simulink subsystem "MPC6_nlpsol"  (R2022b)
settings: Solver=VariableStepAuto  StartTime=0.0  StopTime=10.0  RelTol=1e-3
undefined symbols (not defined in the file): param_global, param_MPC6, param_robot, param_weight_init
settings Model: Creator=emu  LastModifiedBy=emu
settings OptimizationCC: ReuseModelBlockBuffer=on

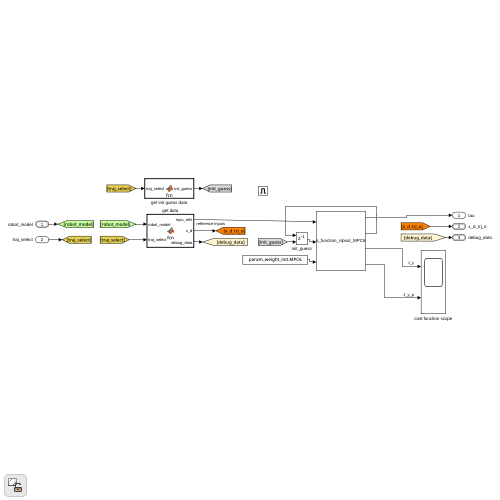
[thumbnail: Simulink's stored preview of the top-level diagram]
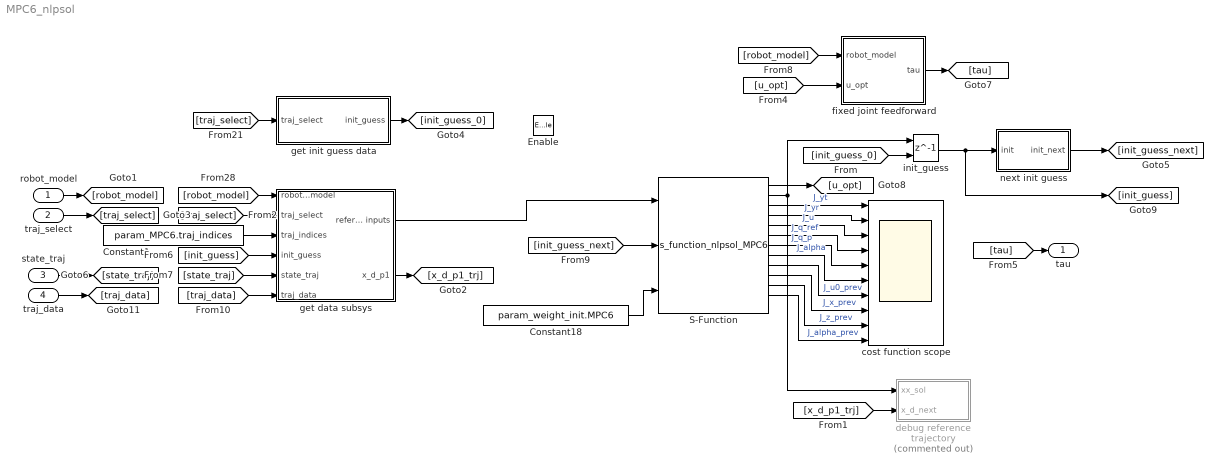
== system MPC6_nlpsol ==
  robot_model : Inport  OutDataTypeStr=Bus: robot_model
  traj_select : Inport  Port=2
  state_traj : Inport  Port=3  OutDataTypeStr=Bus: state_traj_bus
  traj_data : Inport  Port=4  OutDataTypeStr=Bus: traj_data_bus
  Enable : EnablePort
  Constant1 : Constant  Value=param_MPC6.traj_indices
  Constant18 : Constant  Value=param_weight_init.MPC6  VectorParams1D=off
  S-Function : S-Function  FunctionName=s_function_nlpsol_MPC6  Parameters='s_functions/fr3_no_hand_6dof/MPC6.casadi', 'MPC6'  SFunctionModules='MPC6'  SFunctionDeploymentMode=off  EnableBusSupport=off
  cost function scope : Scope  NumInputPorts=10
  debug reference trajectory : Subsystem  Commented=on
  fixed joint feedforward : MATLAB Function  TreatAsAtomicUnit=on
  get data subsys : Subsystem
  get init guess data : MATLAB Function  TreatAsAtomicUnit=on
  init_guess : Delay  DelayLength=1  InitialConditionSource=Input port  InitialCondition=1
      settings: InputPortMap=u0,p4
  next init guess : MATLAB Function  TreatAsAtomicUnit=on
  tau : Outport
  wires:
  S-Function/12 -> cost function scope/10  "J_alpha_prev"
  S-Function/7 -> cost function scope/5  "J_q_p"
  S-Function/10 -> cost function scope/8  "J_x_prev"
  S-Function/3 -> cost function scope/1  "J_yt"
  S-Function/6 -> cost function scope/4  "J_q_ref"
  S-Function/4 -> cost function scope/2  "J_yr"
  S-Function/5 -> cost function scope/3  "J_u"
  S-Function/11 -> cost function scope/9  "J_z_prev"
  S-Function/9 -> cost function scope/7  "J_u0_prev"
  S-Function/8 -> cost function scope/6  "J_alpha"
  next init guess/1(init_next) -> [init_guess_next]
  [init_guess_0] -> init_guess/2
  get init guess data/1(init_guess) -> [init_guess_0]
  S-Function/2 -> init_guess/1, debug reference trajectory/1(xx_sol)
  [traj_select] -> get init guess data/1(traj_select)
  traj_select/1 -> [traj_select]
  robot_model/1 -> [robot_model]
  Constant18/1 -> S-Function/3
  [x_d_p1_trj] -> debug reference trajectory/2(x_d_next)
  [robot_model] -> get data subsys/1(robot_model)
  [traj_select] -> get data subsys/2(traj_select)
  Constant1/1 -> get data subsys/3(traj_indices)
  get data subsys/1(reference inputs) -> S-Function/1
  get data subsys/2(x_d_p1) -> [x_d_p1_trj]
  state_traj/1 -> [state_traj]
  [state_traj] -> get data subsys/5(state_traj)
  fixed joint feedforward/1(tau) -> [tau]
  [robot_model] -> fixed joint feedforward/1(robot_model)
  [u_opt] -> fixed joint feedforward/2(u_opt)
  S-Function/1 -> [u_opt]
  [tau] -> tau/1
  init_guess/1 -> next init guess/1(init), [init_guess]
  [init_guess] -> get data subsys/4(init_guess)
  [init_guess_next] -> S-Function/2
  traj_data/1 -> [traj_data]
  [traj_data] -> get data subsys/6(traj_data)

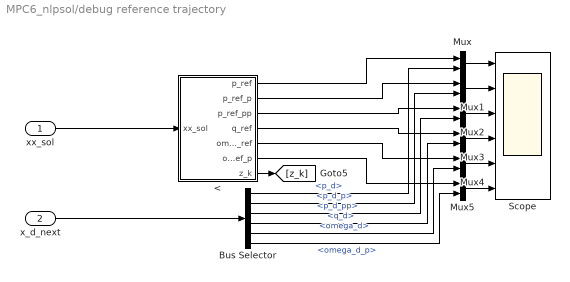
== system MPC6_nlpsol/debug reference trajectory ==
  xx_sol : Inport
  x_d_next : Inport  Port=2  OutDataTypeStr=Bus: x_d
  < : MATLAB Function  TreatAsAtomicUnit=on
  Bus Selector : BusSelector  OutputSignals=p_d,p_d_p,p_d_pp,q_d,omega_d,omega_d_p
  Mux{,1..5} (6 alike) : Mux  Inputs=2
  Scope : Scope  NumInputPorts=6
  wires:
  Mux1/1 -> Scope/2
  </3(p_ref_pp) -> Mux2/1
  Mux5/1 -> Scope/6
  Bus Selector/1 -> Mux/2  "<p_d>"
  Mux3/1 -> Scope/4
  Mux2/1 -> Scope/3
  Bus Selector/6 -> Mux5/2  "<omega_d_p>"
  </4(q_ref) -> Mux3/1
  Bus Selector/2 -> Mux1/2  "<p_d_p>"
  x_d_next/1 -> Bus Selector/1
  Mux/1 -> Scope/1
  </6(omega_ref_p) -> Mux5/1
  Bus Selector/4 -> Mux3/2  "<q_d>"
  </2(p_ref_p) -> Mux1/1
  </7(z_k) -> [z_k]
  </1(p_ref) -> Mux/1
  Bus Selector/5 -> Mux4/2  "<omega_d>"
  xx_sol/1 -> </1(xx_sol)
  </5(omega_ref) -> Mux4/1
  Bus Selector/3 -> Mux2/2  "<p_d_pp>"
  Mux4/1 -> Scope/5

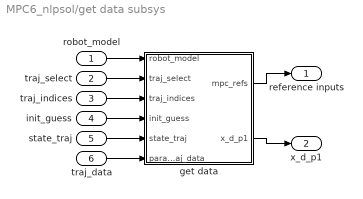
== system MPC6_nlpsol/get data subsys ==
  robot_model : Inport  OutDataTypeStr=Bus: robot_model
  traj_select : Inport  Port=2
  traj_indices : Inport  Port=3
  init_guess : Inport  Port=4
  state_traj : Inport  Port=5  OutDataTypeStr=Bus: state_traj_bus
  traj_data : Inport  Port=6  OutDataTypeStr=Bus: traj_data_bus
  get data : MATLAB Function  TreatAsAtomicUnit=on
  reference inputs : Outport
  x_d_p1 : Outport  Port=2  OutDataTypeStr=Bus: x_d
  wires:
  traj_data/1 -> get data/6(param_traj_data)
  init_guess/1 -> get data/4(init_guess)
  state_traj/1 -> get data/5(state_traj)
  traj_indices/1 -> get data/3(traj_indices)
  get data/1(mpc_refs) -> reference inputs/1
  robot_model/1 -> get data/1(robot_model)
  get data/2(x_d_p1) -> x_d_p1/1
  traj_select/1 -> get data/2(traj_select)

== matlab function MPC6_nlpsol/fixed joint feedforward ==
  data: robot_model input Bus: robot_model; tau output; u_opt input; param_robot parameter
function  tau = fcn(robot_model, u_opt, param_robot)

n = param_robot.n_DOF;

if size(u_opt, 2) ~= 0 && size(u_opt, 1) ~= 1
    n_indices = param_robot.n_indices;
    n_red = param_robot.n_red;

    tau_red = u_opt(1:n_red);
    %q_d_pp = u_opt(1+n_red:2*n_red);

    M = robot_model.M;      % inertia matrix
    g = robot_model.g;
    C_rnea = robot_model.C_rnea; % C_rnea(q, q_p) = C(q, q_p)q_p + g(q) = n(q, q_p)

    Cqp = C_rnea - g;
    M_red = M(n_indices, n_indices);

    %q_pp = zeros(n,1);
    %q_pp(n_indices) = q_d_pp;

    q_pp_red = M_red\(tau_red - Cqp(n_indices)); % gravity is ignored here
    q_pp = zeros(n, 1);
    q_pp(n_indices) = q_pp_red;

    tau = M*q_pp + Cqp;
else
    tau = zeros(n,1);
end

== matlab function MPC6_nlpsol/debug reference trajectory/< ==
  data: xx_sol input; p_ref output; param_MPC6 parameter; p_ref_p output; p_ref_pp output; q_ref output; omega_ref output; omega_ref_p output; z_k output
function [p_ref, p_ref_p, p_ref_pp, q_ref, omega_ref, omega_ref_p, z_k] = fcn(xx_sol, param_MPC6)

if ~isscalar(xx_sol)
    param_MPC = param_MPC6;
    
    zt_indices = param_MPC.zt;
    zt_dim = param_MPC.zt_dim;

    alphat_indices = param_MPC.alphat;
    alphat_dim = param_MPC.alphat_dim;
    
    zr_indices = param_MPC.zr;
    zr_dim_indices = param_MPC.zr_dim;

    alphar_indices = param_MPC.alphar;
    alphar_dim = param_MPC.alphar_dim;

    zt = reshape(xx_sol(zt_indices), zt_dim);
    alphat = reshape(xx_sol(alphat_indices), alphat_dim);
    zr = reshape(xx_sol(zr_indices), zr_dim_indices);
    alphar = reshape(xx_sol(alphar_indices), alphar_dim);
    p_ref = zt(1:3, 1 + (1));
    p_ref_p = zt(4:6, 1 + (1));
    p_ref_pp = alphat(1:3, 1 + (1));
    
    q_ref = zr(1:4, 1 + (1));
    omega_ref = zr(5:7, 1 + (1));
    omega_ref_p = alphar(1:3, 1 + (1));
    
    z_k = [p_ref; p_ref_p; q_ref; omega_ref];
else
    p_ref = zeros(3,1);
    p_ref_p = zeros(3,1);
    p_ref_pp = zeros(3,1);
    
    q_ref = zeros(4,1);
    omega_ref = zeros(3,1);
    omega_ref_p = zeros(3,1);
    
    z_k = [p_ref; p_ref_p; q_ref; omega_ref];
end

== matlab function MPC6_nlpsol/get data subsys/get data ==
  settings: updateMethod=DISCRETE  sampleTime=param_global.Ta
  data: mpc_refs output; robot_model input Bus: robot_model; traj_select input; traj_indices input; init_guess input; state_traj input Bus: state_traj_bus; x_d_p1 output Bus: x_d; param_robot parameter; param_traj_data input
function [mpc_refs, x_d_p1] = fcn(robot_model, traj_select, traj_indices, init_guess, state_traj, param_robot, param_traj_data)
persistent cnt;
persistent run_flag;

if(isempty(cnt))
    cnt = 1;
    run_flag = 0;
end

n_red = param_robot.n_red;
n_indices = param_robot.n_indices;
yt_indices = param_robot.yt_indices;
yr_indices = param_robot.yr_indices;
traj_indices = traj_indices + (cnt-1);
N_MPC = length(traj_indices)-1;

% Parameters
q    = robot_model.q;      % generalized coordinates
q_p  = robot_model.q_p;  % time derivative of generalized coordinates

x_k = [q(n_indices);q_p(n_indices)];

% Assemble vector of recieved output measurements
p_d     = param_traj_data.p_d(   1:3, traj_indices, traj_select);
p_d_p     = param_traj_data.p_d_p(   1:3, traj_indices, traj_select);
p_d_pp     = param_traj_data.p_d_pp(   1:3, traj_indices, traj_select);

q_d    = param_traj_data.q_d(       1:4, traj_indices, traj_select);
%q_d_p  = param_traj_data.q_d_p(     1:4, traj_indices, traj_select);
%q_d_pp = param_traj_data.q_d_pp(    1:4, traj_indices, traj_select);

omega_d   = param_traj_data.omega_d(  1:3, traj_indices, traj_select);
omega_d_p = param_traj_data.omega_d_p(1:3, traj_indices, traj_select);

alpha_d    = param_traj_data.alpha_d(           :, traj_indices, traj_select);
alpha_d_p  = param_traj_data.alpha_d_p(         :, traj_indices, traj_select);
alpha_d_pp = param_traj_data.alpha_d_pp(        :, traj_indices, traj_select);
rot_ax_d   = param_traj_data.rot_ax_d(          :, traj_indices, traj_select);
alpha_d_offset = param_traj_data.alpha_d_offset(:, traj_indices, traj_select);
q_d_rel = param_traj_data.q_d_rel(              :, traj_indices, traj_select);

y_d = [p_d; q_d];
y_d_p = [p_d_p; omega_d];
y_d_pp = [p_d_pp; omega_d_p];

%if(cnt == 1)
%    if(~isempty(yt_indices) && isempty(yr_indices))
%        z_k = [y_d(yt_indices,1); y_d_p(yt_indices,1)]; % q_d_0, omega_d_0
%    elseif(isempty(yt_indices) && ~isempty(yr_indices))
%        z_k = [y_d(4:7,1); y_d_p(4:6,1)]; % q_d_0, omega_d_0
%    elseif(~isempty(yt_indices) && ~isempty(yr_indices))
%        z_k = [y_d(yt_indices,1); y_d_p(yt_indices,1); y_d(4:7,1); y_d_p(4:6,1)]; % p_d_0, q_d_0, p_d_p_0, omega_d_0
%    end
%else
    N_u = n_red*N_MPC;
    N_x = 2*n_red * (N_MPC+1);
    N_z0 = 2*numel(yt_indices)+8;
    z_k = init_guess(1+N_u+N_x+N_z0 : N_u+N_x+2*N_z0); % use z1 as next z0
%end

N_z = N_z0 * (N_MPC+1);
N_alpha = (4+numel(yt_indices))* (N_MPC+1);

%% Reference out
xx_prev = init_guess(1:N_u+N_x+N_z+N_alpha); % = u_prev, x_prev, z_prev, alpha_prev
mpc_refs = [x_k(:); z_k(:); y_d(:); y_d_p(:); y_d_pp(:); xx_prev(:)];

%% NEXT REFERENCE TRAJECTORY OUT
x_d_p1.p_d       = param_traj_data.p_d(1:3, cnt+1 , traj_select);    %y0
x_d_p1.p_d_p     = param_traj_data.p_d_p(1:3, cnt+1 , traj_select);  %y0p
x_d_p1.p_d_pp    = param_traj_data.p_d_pp(1:3, cnt+1 , traj_select); %y0pp
x_d_p1.Phi_d     = param_traj_data.Phi_d(:, cnt+1 , traj_select);
x_d_p1.Phi_d_p   = param_traj_data.Phi_d_p(:, cnt+1, traj_select);
x_d_p1.Phi_d_pp  = param_traj_data.Phi_d_pp(:,cnt+1, traj_select);
x_d_p1.R_d       = param_traj_data.R_d(:,:, cnt+1, traj_select);
x_d_p1.q_d       = q_d(1:4, 2);
x_d_p1.q_d_p     = param_traj_data.q_d_p(1:4, cnt+1, traj_select);
x_d_p1.q_d_pp    = param_traj_data.q_d_pp(1:4, cnt+1, traj_select);
x_d_p1.omega_d   = omega_d(1:3, 2);
x_d_p1.omega_d_p = omega_d_p(1:3, 2);
x_d_p1.alpha_d    = alpha_d(:, 2);
x_d_p1.alpha_d_p  = alpha_d_p(:, 2);
x_d_p1.alpha_d_pp = alpha_d_pp(:, 2);
x_d_p1.rot_ax_d   = rot_ax_d(:, 2);
x_d_p1.alpha_d_offset = alpha_d_offset(:, 2);
x_d_p1.q_d_rel = q_d_rel(:, 2);

[run_flag, cnt] = update_traj_cnt(state_traj, run_flag, cnt, param_traj_data.N);

== matlab function MPC6_nlpsol/get init guess data ==
  data: traj_select input; param_MPC6_init_guess parameter; init_guess output
function init_guess   = fcn(traj_select, param_MPC6_init_guess)

%init_guess = param_MPC6_init_guess.init_guess(1,:);
init_guess = param_MPC6_init_guess.init_guess(traj_select,:);

== matlab function MPC6_nlpsol/next init guess ==
  data: init input; init_next output; param_MPC6 parameter; param_robot parameter; param_global parameter
function init_next = fcn(init, param_MPC6, param_robot, param_global)
param_MPC = param_MPC6;

Ta = param_global.Ta;
dt_arr = param_MPC.int_times;
N_MPC = param_MPC.N;
n_red = param_robot.n_red;
N_u = n_red * N_MPC;
N_x = (2*n_red)*(N_MPC+1);

yt_indices = param_robot.yt_indices;
yr_indices = param_robot.yr_indices;

n_yt_red = numel(yt_indices);
n_alpha = n_yt_red+3;
n_z = 2*n_yt_red+7;
N_z = n_z*(N_MPC+1);
N_alpha = n_alpha*(N_MPC+1);

N = 0;

u_idx = N + [1:N_u];       N = N + length(u_idx);
u_idx_2d = reshape(u_idx, n_red, N_MPC);
u_idx_2d(:, 1:end-1) = u_idx_2d(:, 2:end);

x_idx = N + [1:N_x];       N = N + length(x_idx);
x_idx_2d = reshape(x_idx, 2*n_red, (N_MPC+1));
x_idx_2d(:, 1:end-1) = x_idx_2d(:, 2:end);

z_idx = N + [1:N_z];       N = N + length(z_idx);
z_idx_2d = reshape(z_idx, n_z, (N_MPC+1));
z_idx_2d(:, 1:end-1) = z_idx_2d(:, 2:end);

alpha_idx = N + [1:N_alpha];       N = N + length(alpha_idx);
alpha_idx_2d = reshape(alpha_idx, n_alpha, (N_MPC+1));
alpha_idx_2d(:, 1:end-1) = alpha_idx_2d(:, 2:end);

%q_idx = N + [1:n_red];     N = N + length(q_idx);
%
%lam_u_idx = N + [1:N_u];   N = N + length(lam_u_idx);
%lam_u_idx_2d = reshape(lam_u_idx, n_red, N_MPC);
%lam_u_idx_2d(:, 1:end-1) = lam_u_idx_2d(:, 2:end);
%
%lam_x_idx = N + [1:N_x];   N = N + length(lam_x_idx);
%lam_x_idx_2d = reshape(lam_x_idx, 2*n_red, (N_MPC+1));
%lam_x_idx_2d(:, 1:end-1) = lam_x_idx_2d(:, 2:end);
%
%lam_q_idx = N + [1:n_red]; N = N + length(lam_q_idx);
%
%lam_g_x_idx = N + [1:N_x]; N = N + length(lam_g_x_idx);
%lam_g_idx_2d = reshape(lam_g_x_idx, 2*n_red, (N_MPC+1));
%lam_g_idx_2d(:, 1:end-1) = lam_g_idx_2d(:, 2:end);
%
%lam_g_q_idx = N + [1:n_red];

x_init = init(x_idx_2d);
u_init = init(u_idx_2d);
z_init = init(z_idx_2d);
alpha_init = init(alpha_idx_2d);

dx = (x_init(:, 2:end) - x_init(:, 1:end-1))./dt_arr;
x_next = x_init(:, 1:end-1) + dx * Ta;

du = (u_init(:, 2:end) - u_init(:, 1:end-1))./dt_arr(1:end-1);
u_next = u_init(:, 1:end-1) + du * Ta;

dz = (z_init(:, 2:end) - z_init(:, 1:end-1))./dt_arr(1:end);
z_next = z_init(:, 1:end-1) + dz * Ta;

dalpha = (alpha_init(:, 2:end) - alpha_init(:, 1:end-1))./dt_arr(1:end);
alpha_next = alpha_init(:, 1:end-1) + dalpha * Ta;

x_idx_m1 = x_idx_2d(:, 1:end-1);
u_idx_m1 = u_idx_2d(:, 1:end-1);
z_idx_m1 = z_idx_2d(:, 1:end-1);
alpha_idx_m1 = alpha_idx_2d(:, 1:end-1);

init_next = init';
%init_next = init([u_idx_2d(:); x_idx_2d(:); q_idx(:); lam_u_idx_2d(:); lam_x_idx_2d(:); lam_q_idx(:); lam_g_idx_2d(:); lam_g_q_idx(:)])';
init_next(x_idx_m1) = x_next;
init_next(u_idx_m1) = u_next;
%init_next(z_idx_m1) = z_next;
%init_next(alpha_idx_m1) = alpha_next;
